simulink model "psbdcvoltage"  (Simulink 6.0)
settings: Solver=ode23s  SolverMode=SingleTasking  StartTime=0.0  StopTime=0.01  RelTol=1e-3  AbsTol=1e-6
libraries: powerlib2 x8
settings Model: Creator=patrice  LastModifiedBy=batserve  ExtModeTrigMode=oneshot  ExtModeArmWhenConnect=off  ExtModeAutoUpdateStatusClock=off
settings DataIOCC: LimitDataPoints=off
settings OptimizationCC: BooleanDataType=off
settings DebuggingCC: SolverPrmCheckMsg=none
settings HardwareCC: TargetUnknown=on
settings RTWCC: TemplateMakefile=grt_unix.tmf

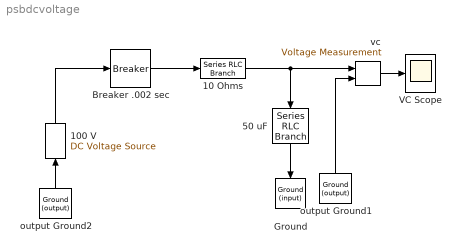
== system psbdcvoltage ==
  10 Ohms : powerlib2/Elements/Series RLC Branch  Tag=PoWeRsYsTeMbLoCk  a=10  b=0  c=inf  mesure=None  PSBOutputType=1
  100 V : powerlib2/Electrical Sources/DC Voltage Source  Tag=PoWeRsYsTeMbLoCk  Orientation=up  V=100  mesure=None  PSBOutputType=1
  50 uF : powerlib2/Elements/Series RLC Branch  Tag=PoWeRsYsTeMbLoCk  Orientation=down  a=0  b=0  c=50e-6  mesure=None  PSBOutputType=1
  Breaker .002 sec : powerlib2/Elements/Breaker  Tag=PoWeRsYsTeMbLoCk  a=0.01  c=0  rs=inf  cs=0  times=[ .002 ]  comext=off  mesure=None  PSBOutputType=1
  Ground : powerlib2/Connectors/Ground (input)  Tag=PoWeRsYsTeMbLoCk  Orientation=down
  VC Scope : Scope
      settings: TickLabels=on  TimeRange=0.01  YMin=-10  YMax=120  DataFormat=Array
  output Ground1 : powerlib2/Connectors/Ground (output)  Tag=PoWeRsYsTeMbLoCk  Orientation=up  PSBOutputType=1
  output Ground2 : powerlib2/Connectors/Ground (output)  Tag=PoWeRsYsTeMbLoCk  Orientation=up  PSBOutputType=1
  vc : powerlib2/Measurements/Voltage Measurement  Tag=PoWeRsYsTeMmEaSuReMeNt  PSBOutputType=0  PSBequivalent=1
  wires:
  100 V/1 -> Breaker .002 sec/1
  Breaker .002 sec/1 -> 10 Ohms/1
  output Ground2/1 -> 100 V/1
  10 Ohms/1 -> vc/1, 50 uF/1
  50 uF/1 -> Ground/1
  vc/1 -> VC Scope/1
  output Ground1/1 -> vc/2
